simulink model "Mason"  (R2015b)
settings: Solver=VariableStepAuto  StartTime=0.0  StopTime=10.0  RelTol=1e-3
values from neighbouring files (symbols this model uses):
  B_m = 3.0e-6    (= 3e-06)    [main.m]    (also in motorselection.m)
  g = 9.8    [main.m]
  J_eff = J_m + J_g + (1./(N.^2)).*(J_T + J_s)    [main.m]    (also in motorselection.m)
  K_T = [0.225, 0.175, 0.125, 0.275]    [main.m]    (also in motorselection.m)
  N = 15    [main.m]
undefined symbols (not defined in the file or in its folder): L, R, r
settings Model: Creator=Matthew Blanchard  LastModifiedBy=Matthew Blanchard

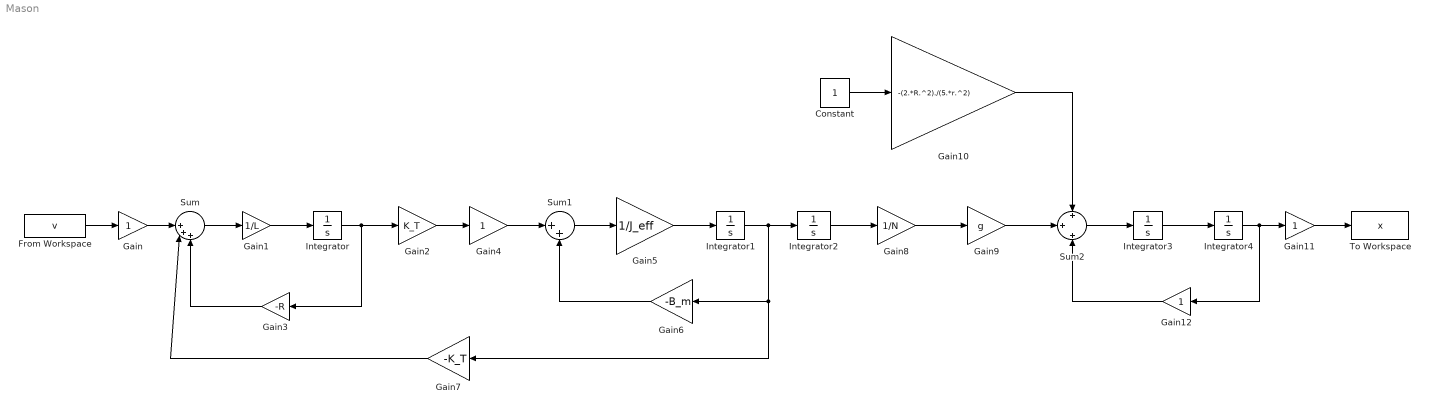
== system Mason ==
  Constant : Constant
  From Workspace : FromWorkspace  VariableName=v  SampleTime=0
  Gain{,4,11..12} (4 alike) : Gain
  Gain1 : Gain  Gain=1/L
  Gain10 : Gain  Gain=-(2.*R.^2)./(5.*r.^2)
  Gain2 : Gain  Gain=K_T
  Gain3 : Gain  Gain=-R
  Gain5 : Gain  Gain=1/J_eff
  Gain6 : Gain  Gain=-B_m
  Gain7 : Gain  Gain=-K_T
  Gain8 : Gain  Gain=1/N
  Gain9 : Gain  Gain=g
  Integrator{,1..4} (5 alike) : Integrator
  Sum : Sum  Inputs=||+++
  Sum1 : Sum  Inputs=|++
  Sum2 : Sum  Inputs=+|+|+
  To Workspace : ToWorkspace  VariableName=x  SaveFormat=Timeseries  SampleTime=-1
  wires:
  Gain/1 -> Sum/1
  From Workspace/1 -> Gain/1
  Sum/1 -> Gain1/1
  Gain1/1 -> Integrator/1
  Integrator/1 -> Gain3/1, Gain2/1
  Gain2/1 -> Gain4/1
  Gain4/1 -> Sum1/1
  Sum1/1 -> Gain5/1
  Gain5/1 -> Integrator1/1
  Integrator1/1 -> Gain7/1, Gain6/1, Integrator2/1
  Gain6/1 -> Sum1/2
  Gain7/1 -> Sum/2
  Gain3/1 -> Sum/3
  Integrator2/1 -> Gain8/1
  Gain8/1 -> Gain9/1
  Gain9/1 -> Sum2/2
  Constant/1 -> Gain10/1
  Gain10/1 -> Sum2/1
  Sum2/1 -> Integrator3/1
  Integrator3/1 -> Integrator4/1
  Integrator4/1 -> Gain12/1, Gain11/1
  Gain12/1 -> Sum2/3
  Gain11/1 -> To Workspace/1
